simulink model "test_adrc"  (R2024a)
settings: Solver=VariableStepAuto  StartTime=0.0  StopTime=100  RelTol=1e-3
libraries: autolibshared x2, simulink x2, vehdynlibtire x1
settings Model: Creator=pair-andres  LastModifiedBy=pair-andres

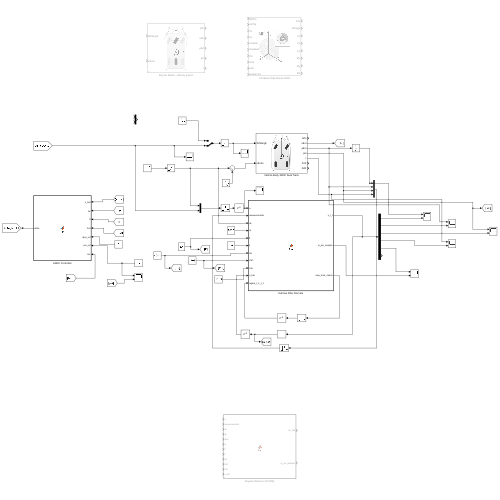
[thumbnail: Simulink's stored preview of the top-level diagram]
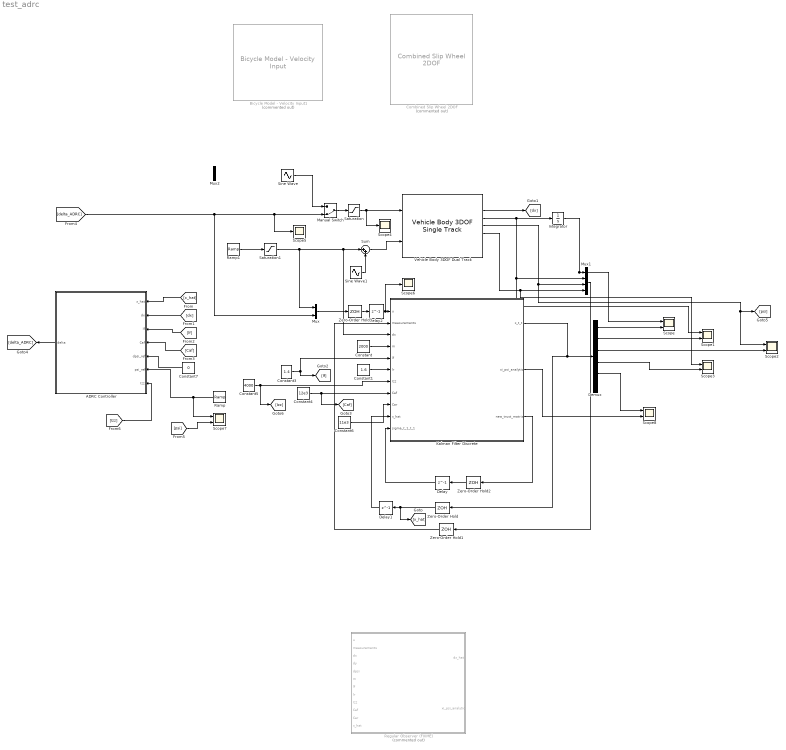
== system test_adrc ==
  ADRC Controller : MATLAB Function  TreatAsAtomicUnit=on
  Bicycle Model - Velocity Input1 : autolibshared/Bicycle Model - Velocity Input  Commented=on  trackMode=Single (bicycle)  inputMode=External longitudinal velocity  frontSteerMode=on  rearSteerMode=off  windMode=off  muMode=off  extFMode=off  extMMode=off  aMode=2  NF=2  NR=2  m=2000  a=1.4  b=1.6  h=0.35  X_o=0  xdot_o=0  CalphaMode=off  sigmaMode=on  w=[1.4,1.4]  Cy_f=12e3  Cy_r=11e3  sigma_f=.1  sigma_r=.1  alpha_f_brk=[-.1 .1]  Cy_f_data=[-9e3 9e3]  alpha_r_brk=[-.1 .1]  Cy_r_data=[-9e3 9e3]  Y_o=0  ydot_o=0  Izz=4000  psi_o=0  r_o=0  Af=2  Cd=.3  Cl=.1  Cpm=.1  beta_w=[0 0.01:0.01:0.3]  Cs=[0 0.01:0.01:0.3]  Cym=[0 1e-6:0.01:0.3]  Pabs=101325  Tair=273  g=9.81  mu=1  xdot_tol=.01  Fznom=5000  Fxtire_sat=1e6  Fytire_sat=1e6  longOff=0  latOff=0  vertOff=0
      settings: LibrarySourceBlock=vehdynlibeom/Bicycle Model - Velocity Input
  Combined Slip Wheel 2DOF : vehdynlibtire/Combined Slip Wheel 2DOF  Commented=on  tireType=External file  BrakeType=Disc  vertType=Magic Formula  plySteer=on  turnslip=on  mu_static=.3  mu_kinetic=.2  disk_abore=.05  Rm=.177  num_pads=2  drum_abore=0.0508  drum_a=0.123  drum_c=0.212  drum_r=0.15  drum_theta1=0  drum_theta2=126  brake_p_bpt=[1 11.4736842105263 21.9473684210526 32.4210526315789 42.8947368421053 53.3684210526316 63.8421052631579 74.3157894736842 84.7894736842105 95.2631578947368 105.736842105263 116.210526315789 126.684210526316 137.157894736842 147.631578947368 158.105263157895 168.578947368421 179.052631578947 189.526315789474 200]  brake_n_bpt=[0 52.6315789473684 105.263157894737 157.894736842105 210.526315789474 263.157894736842 315.789473684211 368.421052631579 421.052631578947 473.684210526316 526.315789473684 578.947368421053 631.578947368421 684.210526315789 736.842105263158 789.473684210526 842.105263157895 894.736842105263 947.368421052632 1000]  f_brake_t=[43.4900602404453 42.5056030554862 41.5350898940194 40.5780454442085 39.6340111501808 38.7025443887544 37.7832176914519 36.8756180088306 35.9793460143796 35.0940154454303 34.2192524787115 33.3546951383474 32.4999927342521 31.6548053290159 30.8188032315107 29.991666515561 29.1730845621415 28.362755623661 27.5603864089927 26.765691687993;498.991217495636 487.695866636631 476.560505099801 465.579679307235 454.748127933653 444.060772460445 433.51270824929 423.099196101319 412.81565427025 402.657650900201 392.620896861006 382.701238955775 372.894653477208 363.197240090814 353.605216024701 344.114910546964 334.722759712992 325.425301366216 316.219170376863 307.10109410434;954.492374750826 932.886130217776 911.585920305583 890.581313170261 869.862244717126 849.419000532136 829.242198807128 809.322774193808 789.651962526121 770.221286354971 751.0225412433 732.047782773203 713.289314220164 694.739674852612 676.391628817892 658.238154578366 640.272434863842 622.48784710877 604.877954344734 587.436496520688;1409.99353200602 1378.07639379892 1346.61133551136 1315.58294703329 1284.9763615006 1254.77722860383 1224.97168936497 1195.5463522863 1166.48827078199 1137.78492180974 1109.42418562559 1081.39432659063 1053.68397496312 1026.28210961441 999.178041611083 972.361398609768 945.822110014692 919.550392851325 893.536738312604 867.771898937035;1865.49468926121 1823.26665738007 1781.63675071715 1740.58458089631 1700.09047828407 1660.13545667552 1620.7011799228 1581.76993037878 1543.32457903786 1505.34855726451 1467.82583000789 1430.74087040806 1394.07863570608 1357.82454437621 1321.96445440427 1286.48464264117 1251.37178516554 1216.61293859388 1182.19552228048 1148.10730135338;2320.9958465164 2268.45692096121 2216.66216592293 2165.58621475934 2115.20459506754 2065.49368474721 2016.43067048064 1967.99350847127 1920.16088729373 1872.91219271928 1826.22747439018 1780.08741422549 1734.47329644903 1689.36697913801 1644.75086719747 1600.60788667257 1556.92146031639 1513.67548433643 1470.85430624835 1428.44270376973;2776.49700377159 2713.64718454235 2651.68758112871 2590.58784862237 2530.31871185102 2470.8519128189 2412.16016103848 2354.21708656376 2296.9971955496 2240.47582817405 2184.62911877248 2129.43395804292 2074.86795719199 2020.9094138998 1967.53727999066 1914.73113070398 1862.47113546724 1810.73803007899 1759.51309021622 1708.77810618608;3231.99816102678 3158.8374481235 3086.71299633449 3015.58948248539 2945.43282863449 2876.21014089059 2807.88965159632 2740.44066465625 2673.83350380547 2608.03946362882 2543.03076315477 2478.78050186034 2415.26261793494 2352.4518486616 2290.32369278385 2228.85437473538 2168.02081061809 2107.80057582154 2048.17187418409 1989.11350860242;3687.49931828197 3604.02771170464 3521.73841154027 3440.59111634842 3360.54694541796 3281.56836896228 3203.61914215416 3126.66424274874 3050.66981206134 2975.60309908359 2901.43240753707 2828.12704567777 2755.6572786779 2683.9942834234 2613.11010557704 2542.97761876678 2473.57048576894 2404.8631215641 2336.83065815196 2269.44891101877;4143.00047553716 4049.21797528579 3956.76382674606 3865.59275021144 3775.66106220143 3686.92659703397 3599.34863271199 3512.88782084123 3427.50612031721 3343.16673453836 3259.83405191936 3177.4735894952 3096.05193942085 3015.5367181852 2935.89651837023 2857.10086279818 2779.12016091979 2701.92566730665 2625.48944211983 2549.78431343512;4598.50163279235 4494.40823886693 4391.78924195184 4290.59438407447 4190.77517898491 4092.28482510566 3995.07812326983 3899.11139893372 3804.34242857308 3710.73036999313 3618.23569630166 3526.82013331263 3436.44660016381 3347.079152947 3258.68293116342 3171.22410682959 3084.66983607064 2998.98821304921 2914.1482260877 2830.11971585147;5054.00279004754 4939.59850244808 4826.81465715762 4715.59601793749 4605.88929576838 4497.64305317735 4390.80761382767 4285.3349770262 4181.17873682896 4078.2940054479 3976.63734068395 3876.16667713006 3776.84126090677 3678.62158770879 3581.46934395661 3485.34735086099 ...(+2764 chars)]  tireParamSet=vdynPassCar.mat  PRESMAX=1000000  PRESMIN=10000  FZMAX=28000  FZMIN=100  VXLOW=1  KPUMAX=1.5  KPUMIN=-1.5  ALPMAX=1.5  ALPMIN=-1.5  CAMMAX=0.17453  CAMMIN=-0.17453  LONGVL=16.7  FxRelFreqLwrLim=200*pi  FyRelFreqLwrLim=200*pi  MyRelFreqLwrLim=100*pi  omegao=0  br=1e-3  UNLOADED_RADIUS=0.5132  NOMPRES=793000  FNOMIN=14000  WIDTH=0.295  RIM_RADIUS=0.28575  MASS=54.96  IYY=10.664  GRAVITY=-9.81  zo=0  zdoto=0  BREFF=8.25094594147963  DREFF=0.260468730454265  FREFF=0.0735298544471851  Q_RE0=1.00866439868088  Q_V1=0.000760413786224011  Q_V2=0.0463384792019201  Q_FZ1=0  Q_FZ2=15.6870832810226  Q_FZ3=0  Q_FCX=0.138643970247602  Q_FCY=0.10843499565426  Q_FCY2=-0.465763352339538  PFZ1=0.69958166705601  VERTICAL_STIFFNESS=207885.061134007  VERTICAL_DAMPING=500  BOTTOM_OFFST=.01  BOTTOM_STIFF=2e6  LONGITUDINAL_STIFFNESS=388714.175879854  LATERAL_STIFFNESS=157087.404633332  PCFX1=0.18539229191199  PCFX2=0  PCFX3=0  PCFY1=0.163183345037677  PCFY2=0  PCFY3=0.249094918231954  Q_RA1=0.675942571700787  Q_RA2=0.73800463546164  Q_RB1=1.04487486456705  Q_RB2=-1.191763806629  PCX1=1.58523057950359  PDX1=1.0239116238178  PDX2=-0.0842405110022724  PDX3=0  PEX1=0.110312777158455  PEX2=0.313468516038146  PEX3=0  PEX4=0.0016060905760045  PKX1=21.3872544684023  PKX2=14.0006541873175  PKX3=-0.405326109653452  PHX1=0.000212599305364818  PHX2=0.00115950515263055  PVX1=1.59236164471432e-05  PVX2=0.000104321112127671  PPX1=-0.349461321276586  PPX2=0.387840040616429  PPX3=-0.0969947336569324  PPX4=0.0632271859795801  RBX1=12.7633329850276  RBX2=9.5787123658471  RBX3=0  RCX1=1.02796280922059  REX1=-0.45202516851367  REX2=-0.47304886171176  RHX1=0.000233272373115809  QSX1=-0.00788307788961443  QSX2=0.954629515459396  QSX3=0.0155855777667025  QSX4=0.125904607142414  QSX5=1.01110069703963  QSX6=20.1938577118433  QSX7=0.310818120717083  QSX8=-0.0430823751139655  QSX9=0.636494404888216  QSX10=0.142438060591663  QSX11=0.346766530036373  QSX12=0  QSX13=0  QSX14=0  PPMX1=0  PCY1=1.34299950037631  PDY1=0.878267729082195  PDY2=-0.0644597923147385  PDY3=0  PEY1=-0.809776534470972  PEY2=-0.600180598867198  PEY3=0.0991732552633487  PEY4=-6.5577974035573  PEY5=0  PKY1=-15.5714726518315  PKY2=1.73126522291751  PKY3=0.365349873517229  PKY4=1.98176755955416  PKY5=0  PKY6=-0.884005199550313  PKY7=-0.237259727611847  PHY1=-0.00183370557235628  PHY2=0.00346401302716671  PVY1=-0.00675427560163264  PVY2=0.036379218103843  PVY3=-0.163543984089166  PVY4=-0.491003349625726  PPY1=-0.62059646553185  PPY2=-0.0647824842338686  PPY3=-0.164648843290686  PPY4=0.283193909060098  PPY5=0  RBY1=10.7588809173639  RBY2=7.70420065295029  RBY3=3.40283755070691e-06  RBY4=0  RCY1=1.06691874059059  REY1=0.308244924574305  REY2=7.48775032604508e-06  RHY1=0.0118479204960415  RHY2=7.63650177161071e-06  RVY1=0.0560024425050078  RVY2=7.48487127056197e-06  RVY3=0  RVY4=98.4047026517149  RVY5=2.02759273900054  RVY6=15.7623064923347  QSY1=0.00699077564863536  QSY2=0  QSY3=0.00153535478298811  QSY4=8.55710322455322e-05  QSY5=0  QSY6=0  QSY7=0.89443879773793  QSY8=-0.403227641260894  QBZ1=11.666656027484  QBZ2=-1.30355438574485  QBZ3=0  QBZ4=0.177918305399071  QBZ5=-0.162481135068033  QBZ6=0  QBZ9=30.1445534682089  QBZ10=0  QCZ1=1.29026978207574  QDZ1=0.0886972644991399  QDZ2=-0.0058634820161856  QDZ3=0.3805597481383  QDZ4=0  QDZ6=0.00160914918118959  QDZ7=-0.00211036330862154  QDZ8=-0.13921904912557  QDZ9=0.00816585550028243  QDZ10=0  QDZ11=0  QEZ1=-2.19802254534746  QEZ2=1.01850535789165  QEZ3=0  QEZ4=0.278379679112054  QEZ5=-0.548414722765386  QHZ1=0.00148361198869669  QHZ2=0.00202017567585904  QHZ3=0.240316641332066  QHZ4=-0.210114035738085  PPZ1=-0.443927982388615  PPZ2=0  SSZ1=0.00914999585397887  SSZ2=0.0389830656052735  SSZ3=0  SSZ4=0  PDXP1=0.396718274678791  PDXP2=0  PDXP3=0  PKYP1=1.00587060633573  PDYP1=0.40483048923438  PDYP2=0  PDYP3=0  PDYP4=0  PHYP1=0.992731942067188  PHYP2=0.150352945499914  PHYP3=0  PHYP4=-3.98988682633674  PECP1=0.502379254513503  PECP2=0  QDTP1=10.0178654287947  QCRP1=0.200627747200702  QCRP2=0.0995735881599772  QBRP1=0.0997107127960717  QDRP1=1.01432910167423  QDRP2=0  aMode=2
  Constant : Constant  Value=2000
  Constant1 : Constant  Value=1.6
  Constant3 : Constant  Value=1.4
  Constant4 : Constant  Value=12e3
  Constant5 : Constant  Value=4000
  Constant6 : Constant  Value=11e3
  Constant7 : Constant  Value=0
  Delay : Delay  DelayLength=1  SampleTime=0.01
  Delay1 : Delay  DelayLength=1  SampleTime=0.01
  Delay2 : Delay  DelayLength=1  SampleTime=0.01
  Demux : Demux  Outputs=6
  Integrator : Integrator
  Kalman Filter Discrete : MATLAB Function  TreatAsAtomicUnit=on
  Manual Switch : ManualSwitch  CurrentSetting=0
  Mux : Mux  Inputs=2
  Mux1 : Mux
  Mux2 : Mux  Inputs=2
  Ramp : simulink/Sources/Ramp  slope=0.02  start=0  InitialOutput=0
  Ramp1 : simulink/Sources/Ramp  slope=1  start=0  InitialOutput=10
  Regular Observer (FIXME) : MATLAB Function  Commented=on  TreatAsAtomicUnit=on
  Saturation : Saturate  UpperLimit=0.2  LowerLimit=-0.2
  Saturation1 : Saturate  UpperLimit=100
  Scope{,1..3,7..8} (6 alike) : Scope  NumInputPorts=2
  Scope4 : Scope
  Scope5 : Scope
  Scope6 : Scope
  Sine Wave : Sin  Amplitude=0  Frequency=3  SampleTime=0
  Sine Wave1 : Sin  SampleTime=0
  Sum : Sum  Inputs=|++
  Vehicle Body 3DOF Dual Track : autolibshared/Vehicle Body 3DOF Single Track  trackMode=Dual  inputMode=External longitudinal velocity  frontSteerMode=on  rearSteerMode=off  windMode=off  muMode=off  extFMode=off  extMMode=off  htchFMode=off  htchMMode=off  extXo=off  extpsio=off  extxdoto=off  extro=off  extYo=off  extTamb=off  extydoto=off  aMode=2  NF=2  NR=2  m=2000  a=1.4  b=1.6  h=0.35  dh=1  hh=0.2  X_o=0  xdot_o=0  CalphaMode=off  sigmaMode=on  d=0  hl=0  w=[1.4,1.4]  Cy_f=12e3  Cy_r=11e3  sigma_f=.1  sigma_r=.1  alpha_f_brk=[-.1 .1]  Cy_f_data=[-9e3 9e3]  alpha_r_brk=[-.1 .1]  Cy_r_data=[-9e3 9e3]  Y_o=0  ydot_o=0  Izz=4000  psi_o=0  r_o=0  Af=2  Cd=.3  Cl=.1  Cpm=.1  beta_w=[0 0.01:0.01:0.3]  Cs=[0:0.03:0.9]  Cym=[0 1e-6:0.01:0.3]  Pabs=101325  Tair=273  g=9.81  mu=1  xdot_tol=.01  Fznom=5000  Fxtire_sat=7e4  Fytire_sat=7e4  longOff=0  latOff=0  vertOff=0  wrapAng=off
      settings: LibrarySourceBlock=vehdynlibeom/Vehicle Body 3DOF Dual Track
  Zero-Order Hold{,1..3} (4 alike) : ZeroOrderHold  SampleTime=0.01
  wires:
  Constant/1 -> Kalman Filter Discrete/4(m)
  Vehicle Body 3DOF Dual Track/3 -> Scope1/1, Mux1/2, Integrator/1
  Ramp1/1 -> Saturation1/1
  Sine Wave/1 -> Manual Switch/1
  Vehicle Body 3DOF Dual Track/5 -> Scope3/1, Mux1/4
  Mux/1 -> Zero-Order Hold3/1
  Constant3/1 -> [lf], Kalman Filter Discrete/5(lf)
  Constant4/1 -> [Caf], Kalman Filter Discrete/8(Caf)
  Kalman Filter Discrete/1(x_t_t) -> Zero-Order Hold/1, Demux/1
  Integrator/1 -> Scope/1, Mux1/1
  Vehicle Body 3DOF Dual Track/4 -> [psi], Scope2/1, Mux1/3
  Mux1/1 -> Zero-Order Hold1/1
  Demux/1 -> Scope/2
  Demux/2 -> Scope1/2
  Demux/3 -> Scope2/2
  Demux/4 -> Scope3/2
  Constant1/1 -> Kalman Filter Discrete/6(lr)
  Constant5/1 -> [Izz], Kalman Filter Discrete/7(Izz)
  Constant6/1 -> Kalman Filter Discrete/9(Car)
  Zero-Order Hold/1 -> [x_hat], Delay1/1
  Kalman Filter Discrete/3(new_trust_matrix) -> Zero-Order Hold2/1
  Zero-Order Hold2/1 -> Delay/1
  Zero-Order Hold3/1 -> Delay2/1
  Delay/1 -> Kalman Filter Discrete/11(sigma_t_1_t_1)
  Delay1/1 -> Kalman Filter Discrete/10(x_hat)
  Zero-Order Hold1/1 -> Kalman Filter Discrete/2(measurements)
  [x_hat] -> ADRC Controller/1(x_hat)
  Vehicle Body 3DOF Dual Track/2 -> [dx]
  [dx] -> ADRC Controller/2(dx)
  [lf] -> ADRC Controller/3(lf)
  [Caf] -> ADRC Controller/4(Caf)
  ADRC Controller/1(delta) -> [delta_ADRC]
  Manual Switch/1 -> Saturation/1
  Saturation/1 -> Scope4/1, Vehicle Body 3DOF Dual Track/1
  Constant7/1 -> ADRC Controller/5(dpsi_ref)
  [delta_ADRC] -> Mux/2, Scope5/1, Manual Switch/2
  [psi] -> Scope7/2
  [Izz] -> ADRC Controller/7(Izz)
  Ramp/1 -> Scope7/1, ADRC Controller/6(psi_ref)
  Delay2/1 -> Scope6/1, Kalman Filter Discrete/1(u)
  Demux/5 -> Scope8/1
  Kalman Filter Discrete/2(xi_psi_analytic) -> Scope8/2
  Saturation1/1 -> Sum/1, Kalman Filter Discrete/3(dx), Mux/1
  Sine Wave1/1 -> Sum/2
  Sum/1 -> Vehicle Body 3DOF Dual Track/2

== matlab function test_adrc/Regular Observer (FIXME) ==
  data: u input; measurements input; dx_hat output; dx input; dy input; dpsi input; m input; lf input; lr input; Izz input; Caf input; Car input; x_hat input; xi_psi_analytic output
function [dx_hat, xi_psi_analytic]= fcn(u, measurements, dx, dy, dpsi, m, lf, lr, Izz, Caf, Car, x_hat)

L1 = 38*4; L2 = 39*4; L3 = 40*4; L4 = 37*4;

A_aug = [
    0, 1, 0, 0, 0, 0;
    0, 0, 0, 0, 0, 1;
    0, 0, 0, 1, 0, 0;
    0, 0, 0, 0, 1, 0;
    0, 0, 0, 0, 0, 0;
    0, 0, 0, 0, 0, 0
];

C_aug = [
   eye(4), zeros(4,2);
];

L = [
    L1, 0, 0, 0;
    0, L2, 0, 0;
    0, 0, L3, 0;
    0, 0, 0, L4;
    zeros(2,4)
];


% Build matrix B which depends on state variables and complicated terms:

b21 = 0;
b22 = (1/m) * (2*Caf*dx/(dx+dy+dpsi*lf));

b41 = 0;
b42 = (1/Izz) * (2*lf*Caf*dx/(dx+dy+dpsi*lf));

B = [
    0, 0;
    b21, b22;
    0, 0;
    b41, b42;
    0, 0;
    0, 0
];

Aobs = A_aug - L*C_aug;
Bobs = [B L];
% Cobs = eye(6);
% Dobs = zeros(6,2);

% Build disturbance can we?
xi_psi_analytic = (-(2*lf*Caf*(dy+dpsi*lf)*cos(u(2)))/(dx+dy+dpsi*lf) + (2*lr*Car*(dy-dpsi*lf))/(dx) ) *(1/Izz);



% state is going to be a 6x1 vector 
dx_hat = Aobs*x_hat + Bobs*[u; measurements];

== matlab function test_adrc/Kalman Filter Discrete ==
  data: u input; measurements input; x_t_t output; dx input; m input; lf input; lr input; Izz input; Caf input; Car input; x_hat input size=[6,1]; xi_psi_analytic output; sigma_t_1_t_1 input size=[6,6]; new_trust_matrix output
function [x_t_t, xi_psi_analytic, new_trust_matrix]= fcn(u, measurements, dx, m, lf, lr, Izz, Caf, Car, x_hat, sigma_t_1_t_1)

sigma_y_given_x = eye(4)*0.05; % 4 states in the measurements vector
sigma_x = eye(6)*0.05;

% Retrieve dy, dz from measurements
dy = measurements(2);
dpsi = measurements(4);

T = 0.01; % seconds

A_aug = [
    0, 1, 0, 0, 0, 0;
    0, 0, 0, 0, 0, 1;
    0, 0, 0, 1, 0, 0;
    0, 0, 0, 0, 1, 0;
    0, 0, 0, 0, 0, 0;
    0, 0, 0, 0, 0, 0
];

C_aug = [
   eye(4), zeros(4,2);
];

% DEPRECATED (LUENBERGER OBSERVER)
% L = [
%     L1, 0, 0, 0;
%     0, L2, 0, 0;
%     0, 0, L3, 0;
%     0, 0, 0, L4;
%     zeros(2,4)
% ];


% Build matrix B which depends on state variables and complicated terms:

b21 = 0;
b22 = (1/m) * (2*Caf*dx/(dx+dy+dpsi*lf));

b41 = 0;
b42 = (1/Izz) * (2*lf*Caf*dx/(dx+dy+dpsi*lf));

B_aug = [
    0, 0;
    b21, b22;
    0, 0;
    b41, b42;
    0, 0;
    0, 0
];

% Discretize state-space with Zero Order Hold (ZOH):
Ad = eye(6) + A_aug*T;
Bd = T*B_aug;
Cd = C_aug;

% disp('vx')
% disp(dx)


% Predict (Time Update):
x_t_t_1 = Ad*x_hat + Bd*u;
sigma_t_t_1 = Ad * sigma_t_1_t_1 * Ad' + sigma_x;


% Update (Measurement Update):
Kt = sigma_t_t_1 * C_aug' * inv(C_aug*sigma_t_t_1*C_aug' + sigma_y_given_x);
x_t_t = x_t_t_1 + Kt * (measurements - C_aug*x_t_t_1);
sigma_t_t = sigma_t_t_1 - Kt * C_aug * sigma_t_t_1;

new_trust_matrix = sigma_t_t;



% Cobs = eye(6);
% Dobs = zeros(6,2);

% Build disturbance can we?
xi_psi_analytic = (-(2*lf*Caf*(dy+dpsi*lf)*cos(u(2)))/(dx+dy+dpsi*lf) + (2*lr*Car*(dy-dpsi*lf))/(dx) ) *(1/Izz);

== matlab function test_adrc/ADRC Controller ==
  data: x_hat input; delta output size=[1]; dx input; lf input; Caf input; dpsi_ref input; psi_ref input; Izz input
function delta = fcn(x_hat, dx, lf, Caf, dpsi_ref, psi_ref, Izz)


K1 = 24;
K2 = 80;

dy = x_hat(2);
psi = x_hat(3);
dpsi = x_hat(4);
xi_hat_ddpsi = x_hat(5); 

% ADRC Control Law:
delta = ((dx + dy + dpsi*lf)*Izz / (2*lf*Caf*max(1,dx))) * (-xi_hat_ddpsi + 0 - K1*(dpsi - dpsi_ref) - K2*(psi - psi_ref));
